simulink model "tec_guiti_re"  (R2023b)
settings: Solver=VariableStepAuto  StartTime=0.0  StopTime=15000  RelTol=1e-3
model workspace: external: MATLAB File par.m (data not in the file)
values from neighbouring files (symbols this model uses):
  c_air = rho_air*v_air*cp_air*1e-3    (= 86.3013725)    [par.m]
  c_al_in = rho_al*v_al_in*cp_al*1e-3    (= 1610.40932)    [par.m]
  c_al_out = rho_al*v_al_out*cp_al*1e-3    (= 3789.1984)    [par.m]
  c_foam = rho_foam*v_foam*cp_foam*1e-3    (= 10207.56)    [par.m]
  K = 4*K_guiti    (= 9.6)    [par.m]
  K_al_in = 40    [par.m]
  k_al_out = 40    [par.m]
settings Model: Creator=wangxueli  LastModifiedBy=wangxueli

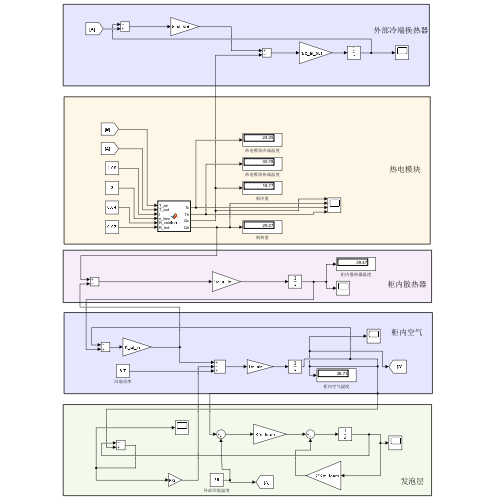
[thumbnail: Simulink's stored preview of the top-level diagram]
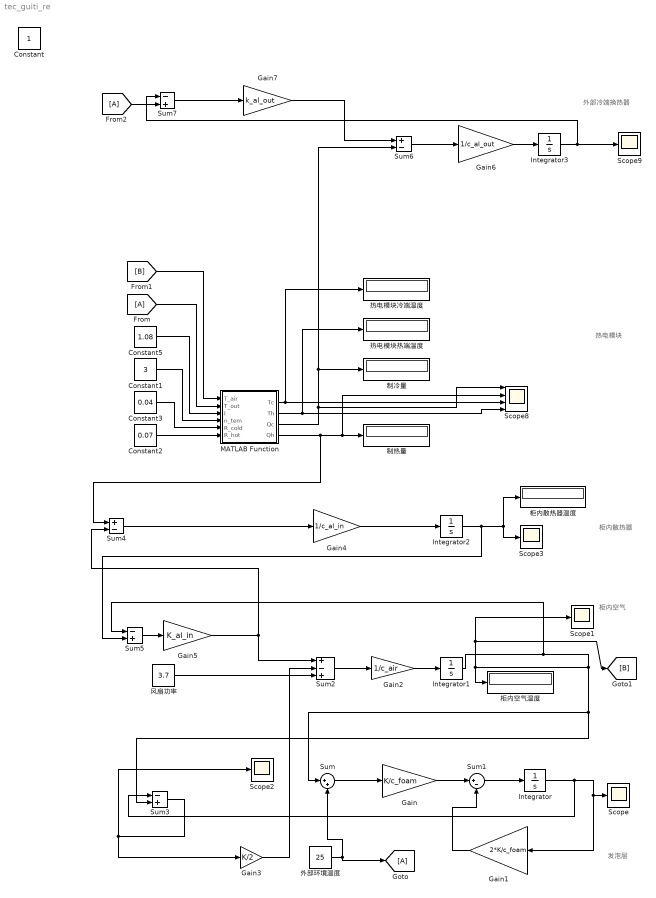
== system tec_guiti_re ==
  note: 热电模块
  note: 外部冷端换热器
  note: 柜内散热器
  note: 柜内空气
  note: 发泡层
  Constant1 : Constant  Value=3
  Constant2 : Constant  Value=0.07
  Constant3 : Constant  Value=0.04
  Constant5 : Constant  Value=1.08
  From : From
  From2 : From
  Gain : Gain  Gain=K/c_foam
  Gain1 : Gain  Gain=2*K/c_foam
  Gain2 : Gain  Gain=1/c_air
  Gain3 : Gain  Gain=K/2
  Gain4 : Gain  Gain=1/c_al_in
  Gain5 : Gain  Gain=K_al_in
  Gain6 : Gain  Gain=1/c_al_out
  Gain7 : Gain  Gain=k_al_out
  Goto : Goto
  Integrator{,1..3} (4 alike) : Integrator  InitialCondition=25
  MATLAB Function : MATLAB Function  TreatAsAtomicUnit=on
  Scope{,1..3,9} (5 alike) : Scope
  Scope8 : Scope  NumInputPorts=4
  Sum : Sum  Inputs=|++
  Sum1 : Sum  Inputs=|+-
  Sum2 : Sum  Inputs=+-+
  Sum3 : Sum  Inputs=-+
  Sum4 : Sum  Inputs=+-
  Sum5 : Sum  Inputs=-+
  Sum6 : Sum  Inputs=+-
  Sum7 : Sum  Inputs=-+
  制冷量 : Display
  制热量 : Display
  外部环境温度 : Constant  Value=25
  柜内散热器温度 : Display
  柜内空气温度 : Display
  热电模块冷端温度 : Display
  热电模块热端温度 : Display
  风扇功率 : Constant  Value=3.7
  Constant : Constant  IOType=siggen
  wires:
  Constant5/1 -> MATLAB Function/3(I)
  Gain4/1 -> Integrator2/1
  From2/1 -> Sum7/2
  MATLAB Function/1(Tc) -> Scope8/3, 热电模块冷端温度/1
  Constant1/1 -> MATLAB Function/4(n_tem)
  Integrator1/1 -> Sum/1, Sum3/2, 柜内空气温度/1, Scope1/1, [B], Sum5/1
  Sum7/1 -> Gain7/1
  [B] -> MATLAB Function/1(T_air)
  Constant2/1 -> MATLAB Function/6(R_hot)
  From/1 -> MATLAB Function/2(T_out)
  Constant3/1 -> MATLAB Function/5(R_cold)
  Integrator2/1 -> Scope3/1, 柜内散热器温度/1, Sum5/2
  Sum5/1 -> Gain5/1
  Integrator3/1 -> Sum7/1, Scope9/1
  风扇功率/1 -> Sum2/3
  Sum3/1 -> Gain3/1, Scope2/1
  Sum1/1 -> Integrator/1
  Gain7/1 -> Sum6/1
  MATLAB Function/3(Qc) -> Sum6/2, 制冷量/1, Scope8/1
  MATLAB Function/4(Qh) -> 制热量/1, Scope8/2, Sum4/1
  Sum4/1 -> Gain4/1
  Gain5/1 -> Sum4/2, Sum2/1
  Gain2/1 -> Integrator1/1
  Gain3/1 -> Sum2/2
  Sum6/1 -> Gain6/1
  Sum2/1 -> Gain2/1
  Gain6/1 -> Integrator3/1
  外部环境温度/1 -> Goto/1, Sum/2
  Sum/1 -> Gain/1
  Gain/1 -> Sum1/1
  Gain1/1 -> Sum1/2
  Integrator/1 -> Gain1/1, Scope/1, Sum3/1
  MATLAB Function/2(Th) -> Scope8/4, 热电模块热端温度/1

== matlab function tec_guiti_re/MATLAB Function ==
  data: T_air input; Tc output; T_out input; I input; Th output; Qc output; Qh output; n_tem input; R_cold input; R_hot input
function [Tc,Th,Qc,Qh] = fcn(T_air,T_out,I,n_tem,R_cold,R_hot)
coder.extrinsic("tec_cal_re");
Tc=0;
Th=0;
Qc=0;
Qh=0;
T0=273.15;
[Tc,Th,Qc,Qh]=tec_cal_re(T_air,T_out,I,n_tem,R_cold,R_hot);
Tc=Tc-273.15;
Th=Th-273.15;
